simulink model "Block"  (R2023b)
settings: Solver=VariableStepAuto  StartTime=0.0  StopTime=30  RelTol=1e-3
values from neighbouring files (symbols this model uses):
  D1 = [5*pi/4,1, 28, 20]    [BaseModel.m]    (also in Block.m = [pi/3, 1, 5, 2]; Model_APF.m = [0,1, 28, 20]; Model_PNG.m = [0, 1,28, 20]; Monte_Carlo.m = [heading_angle, 1.0, D1_y, D1_x])
  D2 = [5*pi/4,1, 27, 35]    [BaseModel.m]    (also in Block.m = [-pi/3, 1, 7, 10]; Model_APF.m = [pi,1, 27, 35]; Model_PNG.m = [pi, 1,27, 35]; Monte_Carlo.m = [-pi/2, 1.0, 0, 0])
  I = [5*pi/4,1.5, 30, 30]    [BaseModel.m]    (also in Block.m = [pi/6, 1.5, 12, 5]; Model_APF.m = [1.5, 30, 30]; Model_PNG.m; Monte_Carlo.m = [5*pi/4, 1.5, 5, 5])
libraries: simulink x2, mcbcontrolslib x2
settings Model: Creator=markzhuang  LastModifiedBy=markzhuang
settings DataIOCC: ReturnWorkspaceOutputs=off

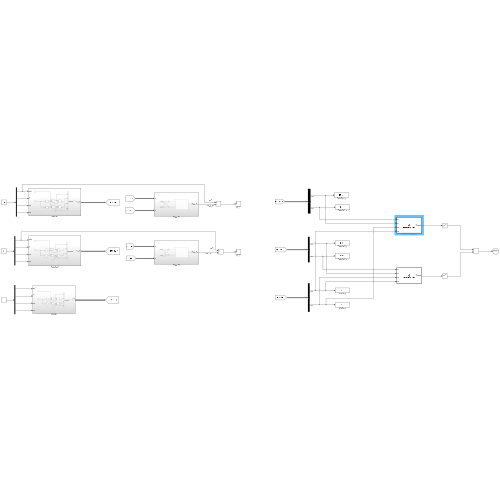
[thumbnail: Simulink's stored preview of the top-level diagram]
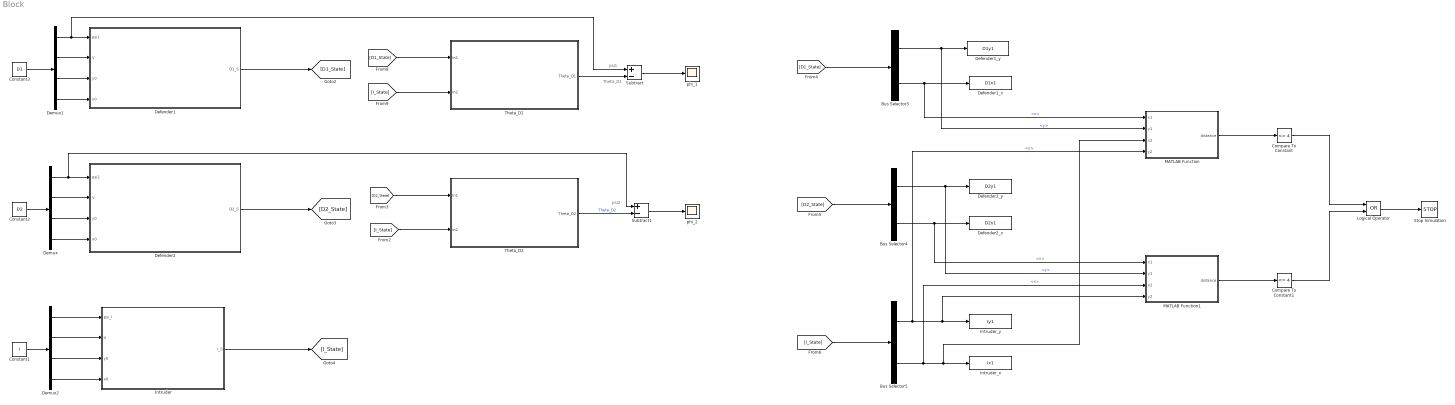
== system Block ==
  note: psi2
  note: Theta_D1
  note: psi1
  Bus Selector3 : BusSelector  OutputSignals=y,x
  Bus Selector4 : BusSelector  OutputSignals=y,x
  Bus Selector5 : BusSelector  OutputSignals=y,x
  Compare To Constant : simulink/Logic and Bit Operations/Compare To Constant  relop=<=  const=4  OutDataTypeStr=boolean
  Compare To Constant1 : simulink/Logic and Bit Operations/Compare To Constant  relop=<=  const=4  OutDataTypeStr=boolean
  Constant1 : Constant  Value=I  VectorParams1D=off
  Constant2 : Constant  Value=D2  VectorParams1D=off
  Constant3 : Constant  Value=D1  VectorParams1D=off
  "Defender1 " : Subsystem
  Defender1_x : ToWorkspace  VariableName=D1x1  SaveFormat=Timeseries  SampleTime=-1
  Defender1_y : ToWorkspace  VariableName=D1y1  SaveFormat=Timeseries  SampleTime=-1
  Defender2 : Subsystem
  Defender2_x : ToWorkspace  VariableName=D2x1  SaveFormat=Timeseries  SampleTime=-1
  Defender2_y : ToWorkspace  VariableName=D2y1  SaveFormat=Timeseries  SampleTime=-1
  Demux : Demux
  Demux1 : Demux
  Demux2 : Demux
  Intruder : Subsystem
  Intruder_x : ToWorkspace  VariableName=Ix1  SaveFormat=Timeseries  SampleTime=-1
  Intruder_y : ToWorkspace  VariableName=Iy1  SaveFormat=Timeseries  SampleTime=-1
  Logical Operator : Logic  Operator=OR  AllPortsSameDT=off  OutDataTypeStr=boolean
  MATLAB Function : MATLAB Function  TreatAsAtomicUnit=on
  MATLAB Function1 : MATLAB Function  TreatAsAtomicUnit=on
  Stop Simulation : Stop
  Subtract : Sum  Inputs=+-
  Subtract1 : Sum  Inputs=+-
  Theta_D1 : Subsystem
  Theta_D2 : Subsystem
  phi_1 : Scope
  phi_2 : Scope
  wires:
  Constant2/1 -> Demux/1
  Constant1/1 -> Demux2/1
  Constant3/1 -> Demux1/1
  "Defender1 "/1(D1_S) -> [D1_State]
  Defender2/1(D2_S) -> [D2_State]
  Intruder/1(I_S) -> [I_State]
  [I_State] -> Bus Selector5/1
  Bus Selector5/1 -> MATLAB Function/4(y2), MATLAB Function1/4(y2), Intruder_y/1  "<y>"
  Bus Selector3/2 -> MATLAB Function/1(x1), Defender1_x/1  "<x>"
  Bus Selector4/1 -> MATLAB Function1/2(y1), Defender2_y/1  "<y>"
  Bus Selector5/2 -> MATLAB Function1/3(x2), MATLAB Function/3(x2), Intruder_x/1  "<x>"
  [D1_State] -> Bus Selector3/1
  [D2_State] -> Bus Selector4/1
  Bus Selector3/1 -> MATLAB Function/2(y1), Defender1_y/1  "<y>"
  Bus Selector4/2 -> MATLAB Function1/1(x1), Defender2_x/1  "<x>"
  [D1_State] -> Theta_D1/1(In1)
  [I_State] -> Theta_D1/2(In2)
  [I_State] -> Theta_D2/2(In2)
  [D2_State] -> Theta_D2/1(In1)
  Theta_D1/1(Theta_D1) -> Subtract/2
  Theta_D2/1(Theta_D2) -> Subtract1/2  "Theta_D2"
  Subtract/1 -> phi_1/1
  Subtract1/1 -> phi_2/1
  MATLAB Function/1(distance) -> Compare To Constant/1
  MATLAB Function1/1(distance) -> Compare To Constant1/1
  Compare To Constant/1 -> Logical Operator/1
  Compare To Constant1/1 -> Logical Operator/2
  Logical Operator/1 -> Stop Simulation/1
  Demux/1 -> Subtract1/1, Defender2/1(psi2)
  Demux/2 -> Defender2/2(V)
  Demux/3 -> Defender2/3(y0)
  Demux/4 -> Defender2/4(x0)
  Demux1/1 -> Subtract/1, "Defender1 "/1(psi1)
  Demux1/2 -> "Defender1 "/2(V)
  Demux1/3 -> "Defender1 "/3(y0)
  Demux1/4 -> "Defender1 "/4(x0)
  Demux2/1 -> Intruder/1(psi_I)
  Demux2/2 -> Intruder/2(V)
  Demux2/3 -> Intruder/3(y0)
  Demux2/4 -> Intruder/4(x0)

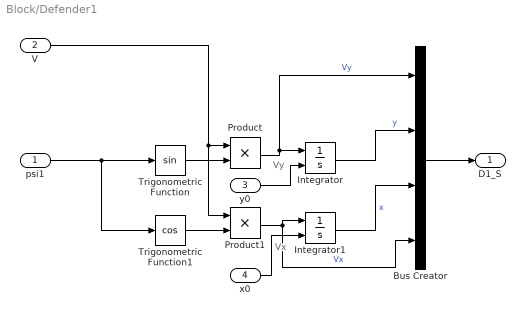
== system Block/Defender1  ==
  note: Vx
  note: Vy
  psi1 : Inport
  V : Inport  Port=2
  y0 : Inport  Port=3
  x0 : Inport  Port=4
  Bus Creator : BusCreator  Inputs=4
  Integrator : Integrator  InitialConditionSource=external
  Integrator1 : Integrator  InitialConditionSource=external
  Product : Product
  Product1 : Product
  Trigonometric Function : Trigonometry
  Trigonometric Function1 : Trigonometry  Operator=cos
  D1_S : Outport
  wires:
  Trigonometric Function/1 -> Product/2
  psi1/1 -> Trigonometric Function1/1, Trigonometric Function/1
  Product1/1 -> Bus Creator/4, Integrator1/1  "Vx"
  V/1 -> Product1/1, Product/1
  Trigonometric Function1/1 -> Product1/2
  y0/1 -> Integrator/2
  x0/1 -> Integrator1/2
  Product/1 -> Bus Creator/1, Integrator/1  "Vy"
  Integrator/1 -> Bus Creator/2  "y"
  Integrator1/1 -> Bus Creator/3  "x"
  Bus Creator/1 -> D1_S/1

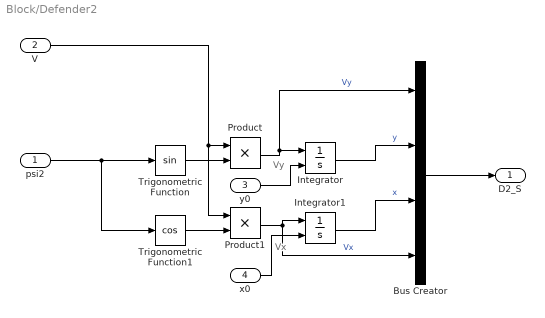
== system Block/Defender2 ==
  note: Vx
  note: Vy
  psi2 : Inport
  V : Inport  Port=2
  y0 : Inport  Port=3
  x0 : Inport  Port=4
  Bus Creator : BusCreator  Inputs=4
  Integrator : Integrator  InitialConditionSource=external
  Integrator1 : Integrator  InitialConditionSource=external
  Product : Product
  Product1 : Product
  Trigonometric Function : Trigonometry
  Trigonometric Function1 : Trigonometry  Operator=cos
  D2_S : Outport
  wires:
  Trigonometric Function/1 -> Product/2
  Product/1 -> Bus Creator/1, Integrator/1  "Vy"
  psi2/1 -> Trigonometric Function1/1, Trigonometric Function/1
  Product1/1 -> Bus Creator/4, Integrator1/1  "Vx"
  V/1 -> Product1/1, Product/1
  Trigonometric Function1/1 -> Product1/2
  Integrator/1 -> Bus Creator/2  "y"
  Integrator1/1 -> Bus Creator/3  "x"
  y0/1 -> Integrator/2
  x0/1 -> Integrator1/2
  Bus Creator/1 -> D2_S/1

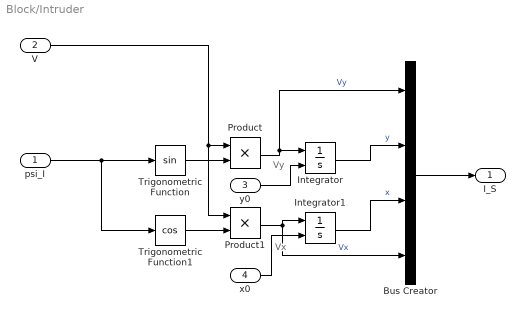
== system Block/Intruder ==
  note: Vx
  note: Vy
  psi_I : Inport
  V : Inport  Port=2
  y0 : Inport  Port=3
  x0 : Inport  Port=4
  Bus Creator : BusCreator  Inputs=4
  Integrator : Integrator  InitialConditionSource=external
  Integrator1 : Integrator  InitialConditionSource=external
  Product : Product
  Product1 : Product
  Trigonometric Function : Trigonometry
  Trigonometric Function1 : Trigonometry  Operator=cos
  I_S : Outport
  wires:
  Trigonometric Function/1 -> Product/2
  Product/1 -> Bus Creator/1, Integrator/1  "Vy"
  psi_I/1 -> Trigonometric Function1/1, Trigonometric Function/1
  Product1/1 -> Bus Creator/4, Integrator1/1  "Vx"
  V/1 -> Product1/1, Product/1
  Trigonometric Function1/1 -> Product1/2
  Integrator/1 -> Bus Creator/2  "y"
  Integrator1/1 -> Bus Creator/3  "x"
  y0/1 -> Integrator/2
  x0/1 -> Integrator1/2
  Bus Creator/1 -> I_S/1

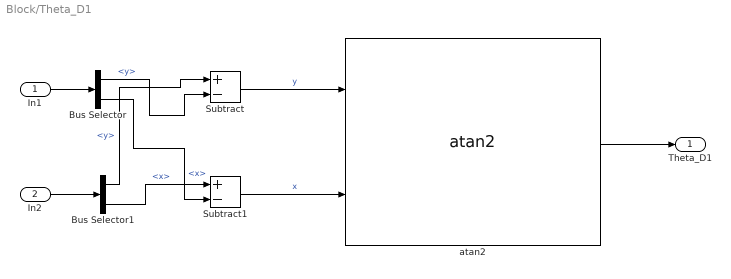
== system Block/Theta_D1 ==
  In1 : Inport
  In2 : Inport  Port=2
  Bus Selector : BusSelector  OutputSignals=y,x
  Bus Selector1 : BusSelector  OutputSignals=y,x
  Subtract : Sum  Inputs=+-
  Subtract1 : Sum  Inputs=+-
  atan2 : mcbcontrolslib/atan2  ApproximationMethod=None  NumberOfIterations=11  NumberOfDataPoints=16  InterpMethod=Flat  outputUnit=Radians  TableDataTypeStr=Inherit: Inherit via input
      settings: LibrarySourceBlock=mcblib/Controls/Math Transforms/atan2
  Theta_D1 : Outport
  wires:
  In1/1 -> Bus Selector/1
  In2/1 -> Bus Selector1/1
  Bus Selector1/1 -> Subtract/1  "<y>"
  Bus Selector/1 -> Subtract/2  "<y>"
  Bus Selector1/2 -> Subtract1/1  "<x>"
  Bus Selector/2 -> Subtract1/2  "<x>"
  Subtract/1 -> atan2/1  "y"
  Subtract1/1 -> atan2/2  "x"
  atan2/1 -> Theta_D1/1

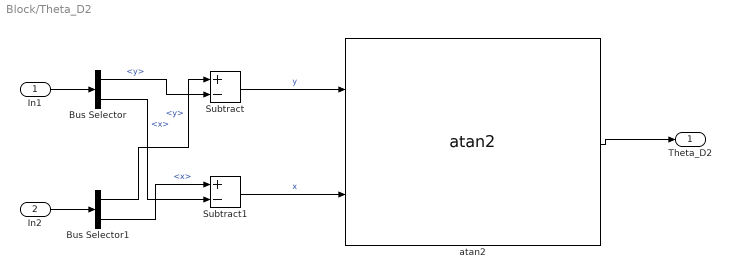
== system Block/Theta_D2 ==
  In1 : Inport
  In2 : Inport  Port=2
  Bus Selector : BusSelector  OutputSignals=y,x
  Bus Selector1 : BusSelector  OutputSignals=y,x
  Subtract : Sum  Inputs=+-
  Subtract1 : Sum  Inputs=+-
  atan2 : mcbcontrolslib/atan2  ApproximationMethod=None  NumberOfIterations=11  NumberOfDataPoints=16  InterpMethod=Flat  outputUnit=Radians  TableDataTypeStr=Inherit: Inherit via input
      settings: LibrarySourceBlock=mcblib/Controls/Math Transforms/atan2
  Theta_D2 : Outport
  wires:
  In1/1 -> Bus Selector/1
  In2/1 -> Bus Selector1/1
  Bus Selector1/1 -> Subtract/1  "<y>"
  Bus Selector/1 -> Subtract/2  "<y>"
  Bus Selector1/2 -> Subtract1/1  "<x>"
  Bus Selector/2 -> Subtract1/2  "<x>"
  Subtract/1 -> atan2/1  "y"
  Subtract1/1 -> atan2/2  "x"
  atan2/1 -> Theta_D2/1

== matlab function Block/MATLAB Function1 ==
  data: x1 input; distance output; y1 input; x2 input; y2 input
function distance = calculateDistance(x1, y1, x2, y2)
    distance = sqrt((x2 - x1)^2 + (y2 - y1)^2);
end

== matlab function Block/MATLAB Function ==
  data: x1 input; distance output; y1 input; x2 input; y2 input
function distance = calculateDistance(x1, y1, x2, y2)
    distance = sqrt((x2 - x1)^2 + (y2 - y1)^2);
end
